simulink model "example"  (R2018a)
settings: Solver=VariableStepAuto  StartTime=0.0  StopTime=inf  RelTol=1e-3
libraries: dspfdesign x8, dspindex x2
settings Model: Creator=bmeat  LastModifiedBy=bmeat

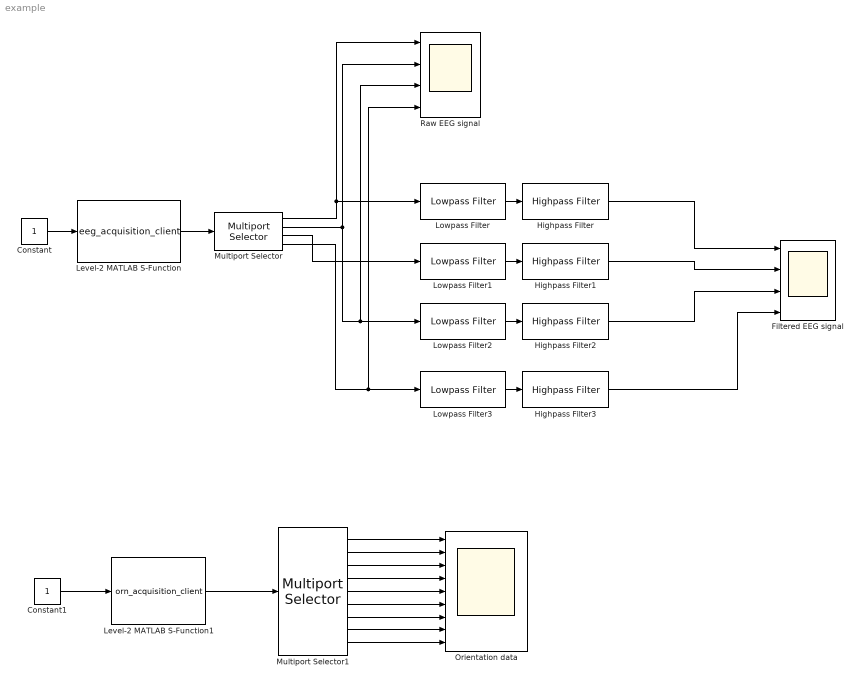
== system example ==
  Constant : Constant  SampleTime=1/250
  Constant1 : Constant  SampleTime=1/23
  Filtered EEG signal : Scope  NumInputPorts=4
  Highpass Filter{,1..3} (4 alike) : dspfdesign/Highpass Filter  FilterType=FIR  DesignForMinimumOrder=on  FilterOrder=50  StopbandFrequency=0.5  PassbandFrequency=1  StopbandAttenuation=60  PassbandRipple=0.1  InheritSampleRate=on  SampleRate=44100  SimulateUsing=Interpreted execution  roundingMode=Floor  coeffsDataTypeStr=fixdt(1,16)
      settings: SourceProductName=DSP System Toolbox
  Level-2 MATLAB S-Function : M-S-Function  FunctionName=eeg_acquisition_client
  Level-2 MATLAB S-Function1 : M-S-Function  FunctionName=orn_acquisition_client
  Lowpass Filter{,1..3} (4 alike) : dspfdesign/Lowpass Filter  FilterType=FIR  DesignForMinimumOrder=on  FilterOrder=50  PassbandFrequency=20  StopbandFrequency=30  PassbandRipple=0.1  StopbandAttenuation=60  InheritSampleRate=on  SampleRate=250  SimulateUsing=Interpreted execution  roundingMode=Floor  coeffsDataTypeStr=fixdt(1,16)
  Multiport Selector : dspindex/Multiport Selector  rowsOrCols=Rows  idxCellArray={1,2,3,4}  idxErrMode=Clip Index
  Multiport Selector1 : dspindex/Multiport Selector  rowsOrCols=Rows  idxCellArray={1,2,3,4,5,6,7,8,9}  idxErrMode=Clip Index
  Orientation data : Scope  NumInputPorts=9
  Raw EEG signal : Scope  NumInputPorts=4
  wires:
  Constant/1 -> Level-2 MATLAB S-Function/1
  Level-2 MATLAB S-Function/1 -> Multiport Selector/1
  Lowpass Filter/1 -> Highpass Filter/1
  Lowpass Filter1/1 -> Highpass Filter1/1
  Lowpass Filter2/1 -> Highpass Filter2/1
  Lowpass Filter3/1 -> Highpass Filter3/1
  Multiport Selector/1 -> Lowpass Filter/1, Raw EEG signal/1
  Multiport Selector/2 -> Lowpass Filter1/1, Raw EEG signal/2
  Multiport Selector/3 -> Raw EEG signal/3, Lowpass Filter2/1
  Multiport Selector/4 -> Raw EEG signal/4, Lowpass Filter3/1
  Highpass Filter/1 -> Filtered EEG signal/1
  Highpass Filter1/1 -> Filtered EEG signal/2
  Highpass Filter2/1 -> Filtered EEG signal/3
  Highpass Filter3/1 -> Filtered EEG signal/4
  Constant1/1 -> Level-2 MATLAB S-Function1/1
  Level-2 MATLAB S-Function1/1 -> Multiport Selector1/1
  Multiport Selector1/1 -> Orientation data/1
  Multiport Selector1/2 -> Orientation data/2
  Multiport Selector1/3 -> Orientation data/3
  Multiport Selector1/4 -> Orientation data/4
  Multiport Selector1/5 -> Orientation data/5
  Multiport Selector1/6 -> Orientation data/6
  Multiport Selector1/7 -> Orientation data/7
  Multiport Selector1/8 -> Orientation data/8
  Multiport Selector1/9 -> Orientation data/9
